simulink model "OpenLoopSimulation"  (R2024b)
settings: Solver=VariableStepAuto  StartTime=0.0  StopTime=100  RelTol=1e-3
undefined symbols (not defined in the file): btm, Jm, Ktm, Kv, Lm, R
settings Model: Creator=mwali  LastModifiedBy=user
settings RTWCC: GPUComputeCapability=3.5

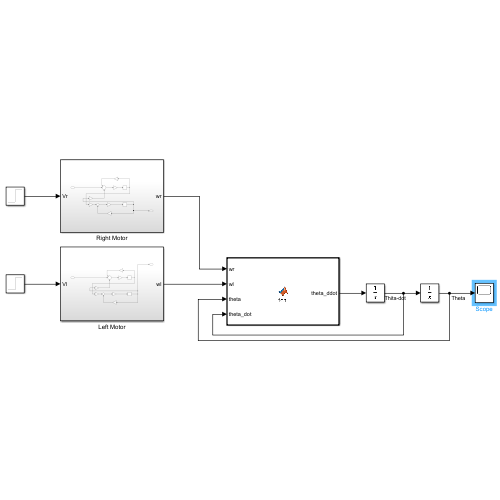
[thumbnail: Simulink's stored preview of the top-level diagram]
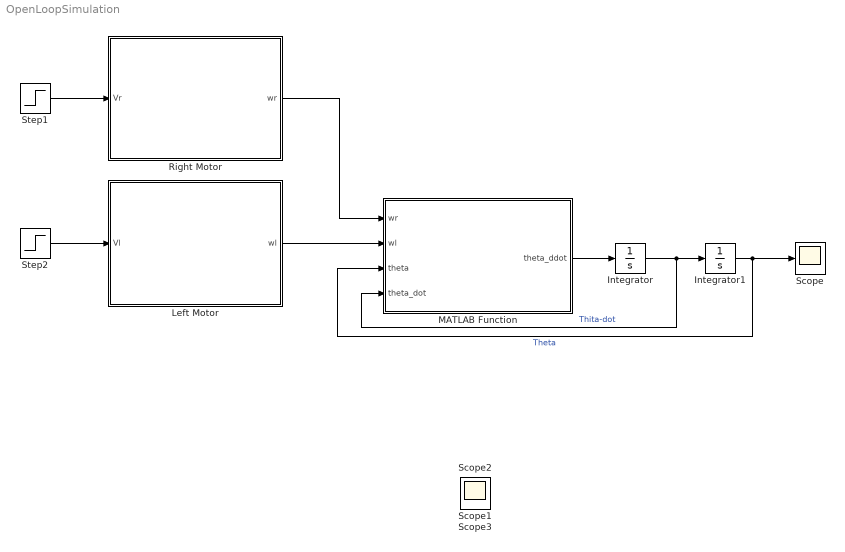
== system OpenLoopSimulation ==
  Integrator : Integrator
  Integrator1 : Integrator
  Left Motor : Subsystem
  MATLAB Function : MATLAB Function  TreatAsAtomicUnit=on
  Right Motor : Subsystem
  Scope{,1..3} (4 alike) : Scope
  Step1 : Step  After=5  SampleTime=0
  Step2 : Step  SampleTime=0
  wires:
  MATLAB Function/1(theta_ddot) -> Integrator/1
  Integrator/1 -> MATLAB Function/4(theta_dot), Integrator1/1  "Thita-dot"
  Integrator1/1 -> MATLAB Function/3(theta), Scope/1  "Theta"
  Step1/1 -> Right Motor/1(Vr)
  Right Motor/1(wr) -> MATLAB Function/1(wr)
  Step2/1 -> Left Motor/1(Vl)
  Left Motor/1(wl) -> MATLAB Function/2(wl)

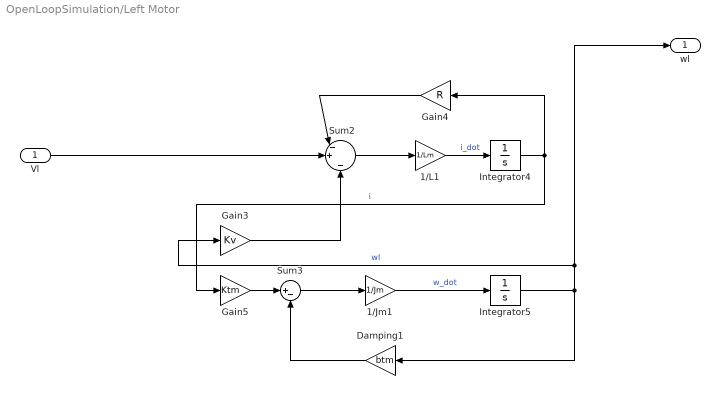
== system OpenLoopSimulation/Left Motor ==
  Vl : Inport
  1/Jm1 : Gain  Gain=1/Jm
  1/L1 : Gain  Gain=1/Lm
  Damping1 : Gain  Gain=btm
  Gain3 : Gain  Gain=Kv
  Gain4 : Gain  Gain=R
  Gain5 : Gain  Gain=Ktm
  Integrator4 : Integrator
  Integrator5 : Integrator
  Sum2 : Sum  Inputs=|-+|-
  Sum3 : Sum  Inputs=|+-
  wl : Outport
  wires:
  Integrator5/1 -> wl/1, Gain3/1, Damping1/1  "wl"
  Sum3/1 -> 1/Jm1/1
  1/L1/1 -> Integrator4/1  "i_dot"
  Damping1/1 -> Sum3/2
  Sum2/1 -> 1/L1/1
  Gain3/1 -> Sum2/3
  1/Jm1/1 -> Integrator5/1  "w_dot"
  Gain5/1 -> Sum3/1
  Integrator4/1 -> Gain5/1, Gain4/1  "i"
  Gain4/1 -> Sum2/1
  Vl/1 -> Sum2/2

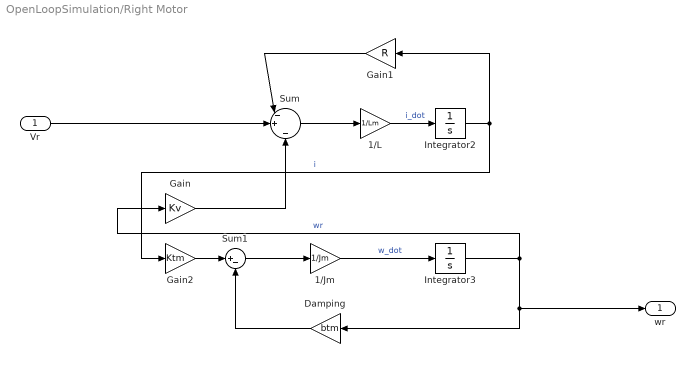
== system OpenLoopSimulation/Right Motor ==
  Vr : Inport
  1/Jm : Gain  Gain=1/Jm
  1/L : Gain  Gain=1/Lm
  Damping : Gain  Gain=btm
  Gain : Gain  Gain=Kv
  Gain1 : Gain  Gain=R
  Gain2 : Gain  Gain=Ktm
  Integrator2 : Integrator
  Integrator3 : Integrator
  Sum : Sum  Inputs=|-+|-
  Sum1 : Sum  Inputs=|+-
  wr : Outport
  wires:
  Gain/1 -> Sum/3
  1/L/1 -> Integrator2/1  "i_dot"
  Sum/1 -> 1/L/1
  Gain1/1 -> Sum/1
  Sum1/1 -> 1/Jm/1
  Damping/1 -> Sum1/2
  Gain2/1 -> Sum1/1
  Integrator3/1 -> Gain/1, wr/1, Damping/1  "wr"
  Integrator2/1 -> Gain2/1, Gain1/1  "i"
  1/Jm/1 -> Integrator3/1  "w_dot"
  Vr/1 -> Sum/2

== matlab function OpenLoopSimulation/MATLAB Function ==
  data: wr input; theta_ddot output; wl input; theta input; theta_dot input
function theta_ddot  = fcn(wr,wl,theta,theta_dot)
   
  L= 600e-3;
  Kt = 100e-6;
  Wo  = 2.0;        
  Lb = 300e-3;
  mb = 75e-3;
  g   = 9.81;
  J = 58.23e-3;
  bt = 10e-3;


    theta_ddot = ((2*L*Kt*Wo * (wr - wl)) - (bt * theta_dot) - ((Lb/2) * mb * g *  theta)) / J;
end
